simulink model "simulink_case4_this"  (R2015b)
settings: Solver=VariableStepAuto  StartTime=0.0  StopTime=10.0  RelTol=1e-3
values from neighbouring files (symbols this model uses):
  kg = b(j)    [Num4s.m]    (also in cont.m; kg_ko.mat = 0.039; num4_45deg.m = b(i); sys4_mass.m)
libraries: simulink x1
settings Model: Creator=guilh_000  LastModifiedBy=guilh_000

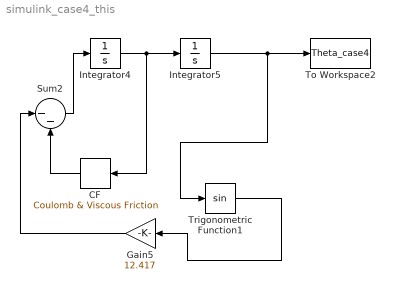
== system simulink_case4_this ==
  CF : simulink/Discontinuities/Coulomb & Viscous Friction  offset=ko  gain=kg
  Gain5 : Gain  Gain=12.417
  Integrator4 : Integrator
  Integrator5 : Integrator  InitialCondition=pi/4
  Sum2 : Sum  Inputs=|--
  To Workspace2 : ToWorkspace  VariableName=Theta_case4  SampleTime=-1
  Trigonometric Function1 : Trigonometry
  wires:
  Integrator4/1 -> CF/1, Integrator5/1
  Sum2/1 -> Integrator4/1
  CF/1 -> Sum2/2
  Gain5/1 -> Sum2/1
  Integrator5/1 -> Trigonometric Function1/1, To Workspace2/1
  Trigonometric Function1/1 -> Gain5/1
